simulink model "ArduinoControl_Monitoring"  (R2019b)
settings: Solver=FixedStepAuto  StartTime=0.0  StopTime=inf  RelTol=1e-3  EnableMultiTasking=on
libraries: arduinolib x4
settings Model: SILPILModeSetting=veronly  ExtModeTrigDuration=2  Creator=FAST  LastModifiedBy=FAST
settings OptimizationCC: EnhancedBackFolding=on  PassReuseOutputArgsAs=Individual arguments  ZeroExternalMemoryAtStartup=off  ZeroInternalMemoryAtStartup=off  MaxStackSize=64  OptimizeBlockOrder=speed  DifferentSizesBufferReuse=on  OptimizationCustomize=off  EfficientTunableParamExpr=on
settings DebuggingCC: ParameterTunabilityLossMsg=error
settings HardwareCC: ProdBitPerInt=16  ProdBitPerPointer=16  ProdBitPerSizeT=16  ProdBitPerPtrDiffT=16  ProdLargestAtomicFloat=None  ProdWordSize=8  ProdHWDeviceType=Atmel->AVR
settings SFSimCC: MATLABDynamicMemAlloc=off
settings RTWCC: SystemTargetFile=ert.tlc  HardwareBoard=Arduino Uno  TLCOptions=-aInlineSetEventsForThisBaseRateFcn=TLC_FALSE -aSuppressMultiTaskScheduler=TLC_FALSE -aRateBasedStepFcn=1  TemplateMakefile=ert_default_tmf  GenerateReport=on  Toolchain=Arduino AVR  BuildConfiguration=Faster Runs  IncludeHyperlinkInReport=on  LaunchReport=on  GenerateTraceInfo=on  GenerateTraceReport=on  GenerateTraceReportSl=on  GenerateTraceReportSf=on  GenerateTraceReportEml=on
settings CodeAppCC: ForceParamTrailComments=on  IgnoreCustomStorageClasses=off  OperatorAnnotations=on  SimulinkDataObjDesc=on  SFDataObjDesc=on  InsertBlockDesc=on
settings ERTTargetCC: SupportContinuousTime=on  SupportVariableSizeSignals=on  ExtModeStaticAllocSize=250

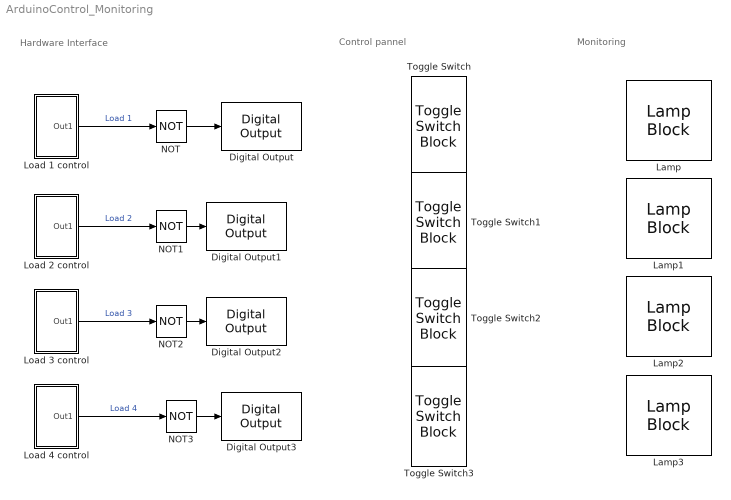
== system ArduinoControl_Monitoring ==
  note: Monitoring
  note: Control pannel
  note: Hardware Interface
  Digital Output : arduinolib/Digital Output  pinNumber=13  blockPlatform=arduino
  Digital Output1 : arduinolib/Digital Output  pinNumber=12  blockPlatform=arduino
  Digital Output2 : arduinolib/Digital Output  pinNumber=11  blockPlatform=arduino
  Digital Output3 : arduinolib/Digital Output  pinNumber=10  blockPlatform=arduino
  Lamp{,1..3} (4 alike) : LampBlock
  Load 1 control : Subsystem
  Load 2 control : Subsystem
  Load 3 control : Subsystem
  Load 4 control : Subsystem
  NOT{,1..3} (4 alike) : Logic  Operator=NOT  IconShape=distinctive  AllPortsSameDT=off  OutDataTypeStr=boolean
  Toggle Switch{,1..3} (4 alike) : ToggleSwitchBlock  LabelPosition=Hide
      settings: Values={{'ON', 'OFF'}, [1 0]}
  wires:
  Load 1 control/1(Out1) -> NOT/1  "Load 1"
  Load 2 control/1(Out1) -> NOT1/1  "Load 2"
  Load 3 control/1(Out1) -> NOT2/1  "Load 3"
  Load 4 control/1(Out1) -> NOT3/1  "Load 4"
  NOT/1 -> Digital Output/1
  NOT1/1 -> Digital Output1/1
  NOT2/1 -> Digital Output2/1
  NOT3/1 -> Digital Output3/1

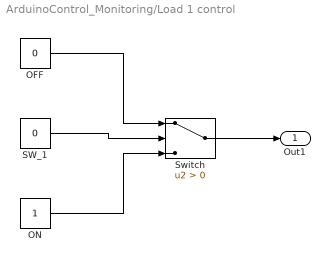
== system ArduinoControl_Monitoring/Load 1 control ==
  OFF : Constant  Value=0
  ON : Constant
  SW_1 : Constant  Value=0
  Switch : Switch  Criteria=u2 > Threshold
  Out1 : Outport
  wires:
  OFF/1 -> Switch/1
  ON/1 -> Switch/3
  SW_1/1 -> Switch/2
  Switch/1 -> Out1/1

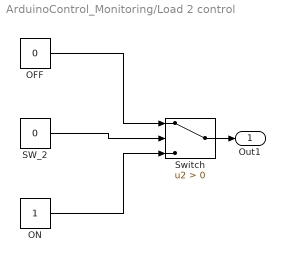
== system ArduinoControl_Monitoring/Load 2 control ==
  OFF : Constant  Value=0
  ON : Constant
  SW_2 : Constant  Value=0
  Switch : Switch  Criteria=u2 > Threshold
  Out1 : Outport
  wires:
  Switch/1 -> Out1/1
  SW_2/1 -> Switch/2
  ON/1 -> Switch/3
  OFF/1 -> Switch/1

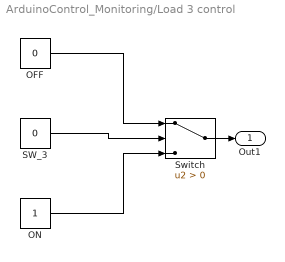
== system ArduinoControl_Monitoring/Load 3 control ==
  OFF : Constant  Value=0
  ON : Constant
  SW_3 : Constant  Value=0
  Switch : Switch  Criteria=u2 > Threshold
  Out1 : Outport
  wires:
  OFF/1 -> Switch/1
  ON/1 -> Switch/3
  SW_3/1 -> Switch/2
  Switch/1 -> Out1/1

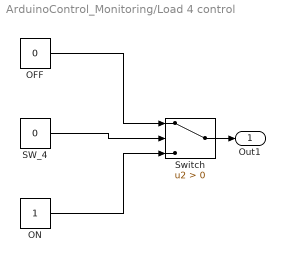
== system ArduinoControl_Monitoring/Load 4 control ==
  OFF : Constant  Value=0
  ON : Constant
  SW_4 : Constant  Value=0
  Switch : Switch  Criteria=u2 > Threshold
  Out1 : Outport
  wires:
  Switch/1 -> Out1/1
  SW_4/1 -> Switch/2
  ON/1 -> Switch/3
  OFF/1 -> Switch/1
